simulink model "CL_Master_Runner"  (R2020b)
settings: configuration reference "VLS_Standard_Configuration" (kept outside this file)
model workspace (MAT data in the model file):
  M_combineLogic = Simulink.Parameter
  M_combineLogic.Value = [0; 1; 0; 1]
  M_combineLogic.DataType = 'boolean'
  M_combineLogic.Dimensions = [4 1]
settings Model: DataDictionary=CL_MasterDD.sldd  EnableAccessToBaseWorkspace=off  Creator=mteama  LastModifiedBy=mtarek-a
settings ConfigSetRef: SourceName=VLS_Standard_Configuration

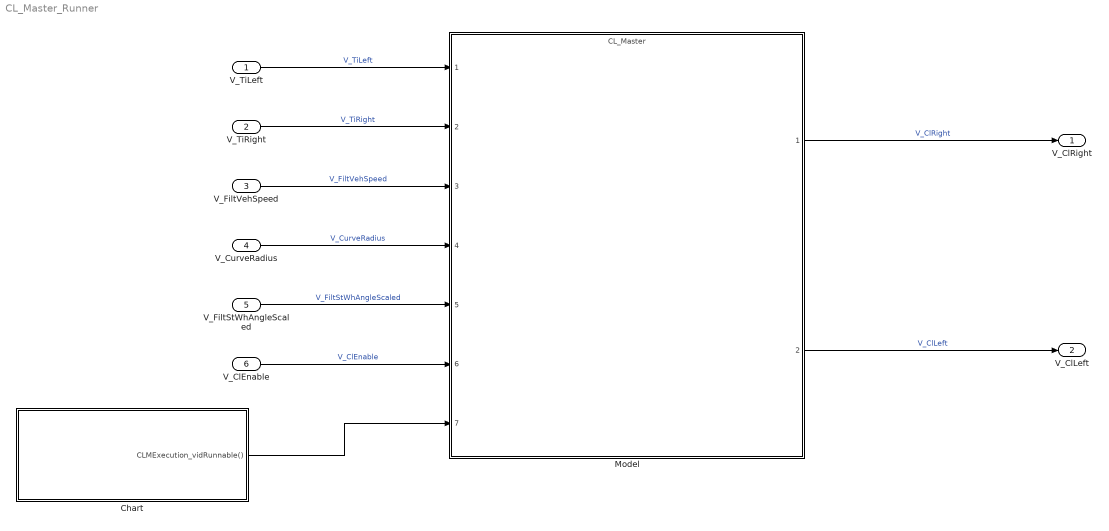
== system CL_Master_Runner ==
  V_TiLeft : Inport
  V_TiRight : Inport  Port=2
  V_FiltVehSpeed : Inport  Port=3
  V_CurveRadius : Inport  Port=4
  V_FiltStWhAngleScaled : Inport  Port=5
  V_ClEnable : Inport  Port=6
  Chart : Stateflow chart  TreatAsAtomicUnit=on
  Model : ModelReference  ModelNameDialog=CL_Master.slx  SimulationMode=Normal  ScheduleRates=on  ModelReferenceVersion=7.159
  V_ClRight : Outport
  V_ClLeft : Outport  Port=2
  wires:
  Model/2 -> V_ClLeft/1  "V_ClLeft"
  Model/1 -> V_ClRight/1  "V_ClRight"
  V_CurveRadius/1 -> Model/4  "V_CurveRadius"
  V_TiLeft/1 -> Model/1  "V_TiLeft"
  V_TiRight/1 -> Model/2  "V_TiRight"
  V_FiltVehSpeed/1 -> Model/3  "V_FiltVehSpeed"
  V_FiltStWhAngleScaled/1 -> Model/5  "V_FiltStWhAngleScaled"
  Chart/1(CLMExecution_vidRunnable()) -> Model/7
  V_ClEnable/1 -> Model/6  "V_ClEnable"

== stateflow chart CL_Master_Runner/Chart ==
  state Scheduler
    on every(1,tick):
    send(CLMExecution_vidRunnable);
  (default) -> Scheduler
  events: CLMExecution_vidRunnable output FUNCTION_CALL_EVENT
